simulink model "s06_sig_template_25"  (R2025b)
settings: Solver=ode4  StopTime=inf  FixedStep=P_sim_dt  EnableMultiTasking=on
InitFcn:
  | s06_data;
values from neighbouring files (symbols this model uses):
  P_c_locate_problist = ones(P_car_cnt, 1, 'single')    [s06_data.m]
  P_display_dt = 50e-3    (= 0.05)    [s06_data.m]
  P_dt = 25e-3    (= 0.025)    [s06_data.m]
  P_p_aMax = 1    [baseline_lqr_script.m]    (also in d71_data.m)
  P_p_Bf = 0.7    [d01_data.m]
  P_p_Br = 0.7    [d01_data.m]
  P_p_Cf = 2    [d01_data.m]
  P_p_Cr = 2    [d01_data.m]
  P_p_delta_max = 21.58/180*pi    (= 0.37664205258)    [d01_data.m]    (also in d71_data.m = 0.383972435439)
  P_p_deltan_max = 1    [d01_data.m]    (also in d71_data.m = 0.93)
  P_p_deltan_min = -P_p_deltan_max    (= -1)    [d01_data.m]    (also in d71_data.m = -0.93)
  P_p_Df = 2    [d01_data.m]
  P_p_Dr = 2.5    [d01_data.m]
  P_p_Ef = -0.1    [d01_data.m]
  P_p_EG = 0    [d01_data.m]    (also in d71_data.m = 0.02)
  P_p_Er = -0.05    [d01_data.m]
  P_p_J = 192e-6    (= 0.000192)    [d01_data.m]    (also in d71_data.m = 3e-06)
  P_p_k = 2.51    [d01_data.m]    (also in d71_data.m = 3.4)
  P_p_kd0 = 0.04    [d71_data.m]
  P_p_kd1 = 0.15    [d71_data.m]
  P_p_l = abs(P_p_frontaxle_1 + P_p_rearaxle_1)    [d01_data.m]    (also in d71_data.m = 0.0325)
  P_p_lf = P_p_frontaxle_1    (= 0.05)    [d01_data.m]    (also in d71_data.m = 0.01625)
  P_p_lr = P_p_rearaxle_1    (= 0.049)    [d01_data.m]    (also in d71_data.m = 0.01625)
  P_p_m = 132e-3    (= 0.132)    [d01_data.m]    (also in d71_data.m = 0.013)
  P_p_T = 316e-3    (= 0.316)    [d01_data.m]    (also in d71_data.m = 0.12)
  P_p_Tt = P_p_uTt + P_p_output_Tt    (= 0.11)    [d01_data.m]    (also in d71_data.m = 0.1)
  P_p_un_max = 1    [d01_data.m]    (also in d71_data.m = 0.2)
  P_p_un_min = -P_p_un_max    (= -1)    [d01_data.m]    (also in d71_data.m = -0.2)
  P_p_vRef = 0.2    [baseline_lqr_script.m]    (also in d71_data.m = 0.15)
  P_p_xvec0 = [ P_p_v0; P_p_s10; P_p_s20; P_p_psi0; 0; 0; 0 ]    [d01_data.m]    (also in d71_data.m)
  P_p_xvec1 = [ P_p_v0; P_p_s11; P_p_s21; P_p_psi1; 0; 0; 0 ]    [d01_data.m]    (also in d71_data.m)
  P_vfilter = single([ 0.0 0.0 ... (first row only)    [s06_data.m]
undefined symbols (not defined in the file or in its folder): CarInputsCmdForward, DiscIntNeverNeededParam, ManeuverTypePark, ManeuverTypePathFollow, mbc_car_display, P_cpseq, P_p, P_track
libraries: vrlib x2
(part 2 of 2)

== matlab function s06_sig_template_25/Car0/Motion Control/Feedback Pathfollowing ==
  data: v_star input; delta_e output; s_star input; psi_star input; s input; psi input; P_p_l parameter
function delta_e = fb_pf(v_star, s_star,psi_star,s,psi,P_p_l)
    %control deviation (see slideset 9 slide 13)
    sc2e=(s(2)-s_star(2))*cos(psi_star)-(s(1)-s_star(1))*sin(psi_star);
    % psi_e = psi - psi_star;
    % if abs(psi_e) < pi
    %     psi_e = -
    psi_e = atan2(sin(psi - psi_star), cos(psi - psi_star)); % wrapped psi_e=psi-psi_star
    
    Tw=0.175; %[s] time constant of pt1 dynamics

    %control law (see slideset 9 slide 20)
    % delta_e = -P_p_l*sc2e/(Tw^2 * v_star^2) - 2*P_p_l*psi_e/(Tw*v_star);

    v_min = 0.05;  % TODO: minimum effective speed, tune this
    v_eff = max(abs(v_star), v_min);

    delta_e = -P_p_l*sc2e/(Tw^2 * v_eff^2) ...
        -2*P_p_l*psi_e/(Tw*v_eff);

== matlab function s06_sig_template_25/Car0/Motion Control/MATLAB Function ==
  data: vRef output; k input; P_dt parameter; P_p_vRef parameter; P_p_aMax parameter
function vRef = generate_vRef(k, P_dt, P_p_vRef, P_p_aMax)
% Generate a discrete ramp speed reference.
%
% Inputs:
%   k          - discrete time index, integer: 0, 1, 2, ...
%   P_dt       - sample time [s]
%   P_p_vRef   - final target speed [m/s]
%   P_p_aMax   - maximum reference acceleration [m/s^2]
%
% Output:
%   vRef       - speed reference [m/s]

t = double(k) * P_dt;

vRef = P_p_aMax * t;

% Hold constant after reaching the target speed
vRef = min(vRef, P_p_vRef);

end

== matlab function s06_sig_template_25/Car0/Motion Control/performance monitor ==
  data: s_car input; psi_car input; SPLINE input; sc2e output; psiError output; progress output; simTime input; reset input; lapCount output; lapDone output; lapTimeLast output; lapIAELast output; lapRMSELast output; lapPsiRMSELast output
function [sc2e, psiError, progress, lapCount, lapDone, ...
          lapTimeLast, lapIAELast, lapRMSELast, ...
          lapPsiRMSELast] = ...
    performance_monitor(s_car, psi_car, SPLINE, simTime, reset)
% PERFORMANCE_MONITOR
% Independent path-following performance measurement.
%
% Inputs
%   s_car    : current vehicle position [x; y]
%   psi_car  : current vehicle heading angle [rad]
%   SPLINE   : MAD76 spline bus signal
%   simTime  : discrete simulation time [s]
%   reset    : reset monitor state
%
% Outputs
%   sc2e            : current signed lateral error [m]
%   psiError        : current wrapped heading error [rad]
%   progress        : accumulated progress in current lap [m]
%   lapCount        : number of completed laps
%   lapDone         : one-sample pulse when a lap is completed
%   lapTimeLast     : duration of last completed lap [s]
%   lapIAELast      : lateral-error IAE over last lap [m*s]
%   lapRMSELast     : lateral-error RMSE over last lap [m]
%   lapPsiRMSELast  : heading-error RMSE over last lap [rad]

persistent initialized
persistent previousArc
persistent previousTime
persistent accumulatedProgress
persistent lapStartTime

persistent lapIAE
persistent lapISE
persistent lapPsiISE

persistent completedLaps

persistent savedLapTime
persistent savedLapIAE
persistent savedLapRMSE
persistent savedLapPsiRMSE

%% Default outputs
sc2e           = 0.0;
psiError       = 0.0;
progress       = 0.0;
lapCount       = uint32(0);
lapDone        = false;
lapTimeLast    = 0.0;
lapIAELast     = 0.0;
lapRMSELast    = 0.0;
lapPsiRMSELast = 0.0;

%% Extract spline data
breakslen = int32(SPLINE.breakslen);
points    = SPLINE.points;
ppcoefs   = SPLINE.coefs;
periodic  = logical(SPLINE.periodic);

if breakslen <= 1
    return;
end

trackLength = double(points(1, breakslen));

if trackLength <= 0
    return;
end

%% Find nearest point on the reference spline
[arcPosition, nearestIndex] = mbc_spline_get_nearest( ...
    breakslen, ...
    points, ...
    ppcoefs, ...
    periodic, ...
    s_car, ...
    int32(1), ...
    breakslen);

%% Evaluate spline at nearest arc-length position
[s_ref, sd_ref, ~, ~] = mbc_ppval( ...
    breakslen, ...
    points(1,:), ...
    ppcoefs, ...
    arcPosition, ...
    nearestIndex);

%% Reference heading
psi_ref = double(atan2(sd_ref(2), sd_ref(1)));

%% Signed lateral error
normal_ref = [-sin(psi_ref);
               cos(psi_ref)];

position_error = ...
    double(s_car(1:2)) - double(s_ref(1:2));

sc2e = normal_ref.' * position_error;

%% Wrapped heading error
% Result is always between -pi and pi.
psiDifference = double(psi_car) - psi_ref;

psiError = atan2( ...
    sin(psiDifference), ...
    cos(psiDifference));

%% Initialization or external reset
if isempty(initialized) || reset
    initialized = true;

    previousArc         = double(arcPosition);
    previousTime        = double(simTime);
    accumulatedProgress = 0.0;
    lapStartTime        = double(simTime);

    lapIAE    = 0.0;
    lapISE    = 0.0;
    lapPsiISE = 0.0;

    completedLaps = uint32(0);

    savedLapTime    = 0.0;
    savedLapIAE     = 0.0;
    savedLapRMSE    = 0.0;
    savedLapPsiRMSE = 0.0;

    progress       = 0.0;
    lapCount       = completedLaps;
    lapTimeLast    = savedLapTime;
    lapIAELast     = savedLapIAE;
    lapRMSELast    = savedLapRMSE;
    lapPsiRMSELast = savedLapPsiRMSE;

    return;
end

%% Time increment
dt = double(simTime) - previousTime;

if dt < 0
    dt = 0.0;
end

%% Unwrap periodic arc-length increment
deltaArc = double(arcPosition) - previousArc;

if periodic
    if deltaArc < -0.5 * trackLength
        % Forward crossing from track end to track beginning
        deltaArc = deltaArc + trackLength;

    elseif deltaArc > 0.5 * trackLength
        % Backward crossing from track beginning to track end
        deltaArc = deltaArc - trackLength;
    end
end

accumulatedProgress = accumulatedProgress + deltaArc;

%% Accumulate error metrics
% Lateral IAE
lapIAE = lapIAE + abs(sc2e) * dt;

% Lateral ISE
lapISE = lapISE + sc2e^2 * dt;

% Heading-error ISE
lapPsiISE = lapPsiISE + psiError^2 * dt;

%% Detect completed lap
if accumulatedProgress >= trackLength
    currentLapTime = double(simTime) - lapStartTime;

    savedLapTime = currentLapTime;
    savedLapIAE  = lapIAE;

    if currentLapTime > 0
        savedLapRMSE = sqrt( ...
            lapISE / currentLapTime);

        savedLapPsiRMSE = sqrt( ...
            lapPsiISE / currentLapTime);
    else
        savedLapRMSE    = 0.0;
        savedLapPsiRMSE = 0.0;
    end

    completedLaps = completedLaps + uint32(1);
    lapDone = true;

    % Preserve progress beyond the finish line
    accumulatedProgress = ...
        accumulatedProgress - trackLength;

    % Start measuring the next lap
    lapStartTime = double(simTime);

    lapIAE    = 0.0;
    lapISE    = 0.0;
    lapPsiISE = 0.0;
end

%% Update persistent states
previousArc  = double(arcPosition);
previousTime = double(simTime);

%% Outputs
progress       = accumulatedProgress;
lapCount       = completedLaps;
lapTimeLast    = savedLapTime;
lapIAELast     = savedLapIAE;
lapRMSELast    = savedLapRMSE;
lapPsiRMSELast = savedLapPsiRMSE;

end

== matlab function s06_sig_template_25/Car0/Motion Control/Discrete-time Handler ==
  data: v input; k output; s input; psi input; v_k output; s_k output; psi_k output; Yp_k output
function [k, v_k, s_k, psi_k, Yp_k] = DiscreteTimeHandler(v, s, psi)

    persistent k_internal % discrete time index

    % initialize only once
    if isempty(k_internal)
        k_internal = -1;
    end

    % upon every incoming sample
    k_internal = k_internal + 1;

    % output
    k = k_internal;
    v_k = v; % this is to make sure the states we use later is consistent with the index
    s_k = s;
    psi_k = psi;

    %% integration for Yp
    persistent Yp_internal
    if isempty(Yp_internal)
        Yp_internal = 0;
    end
    
    Ts = 25e-3; % TODO: find the parameter in data.m
    Yp_internal = Yp_internal + double(v_k)*Ts;
    Yp_k = Yp_internal;

    %% NOTSURE: should we also initialize x0, v0 here? but in our case they
    % are just 0, right?

end

== matlab function s06_sig_template_25/Car0/Motion Control/SampledPositionReference ==
  data: wp input; k input; wp_k output; tE input
function wp_k = SampledPositionReference(wp, k, tE)
    
    Ts = 25e-3; % TODO: I really think we can find this parameter somewhere
    t = k*Ts;
    lap = 0;
    if t>tE
        lap = double(floor(t/tE));
        t = double(mod(t, tE));
    end
    wp_k = wp(6)*t^5 + wp(5)*t^4 + wp(4)*t^3 + wp(3)*t^2 + wp(2)*t + wp(1);
    wp_k = wp_k + lap * 2;
    % c5 = wp(6);
    % c4 = wp(5);
    % c3 = wp(4);
    % wp_k =-0.0008*t^4 + 0.0077 * t^3;
    % wp_k = c4*t^4 + c3*t^3;
    % 
    % if wp_k > 2
    %     wp_k = single(2);
    % end
    
end

== matlab function s06_sig_template_25/Car0/Motion Control/Position Feedforward Controller ==
  data: k input; uvp_k output; wp input; tE input
function uvp_k = PositionFeedFowardControl(k, wp, tE)

% analytical solution for feedforward signal 
% uvp(t) = Tw*wa(t+Tt)+wv(t+Tt)
    Ts = 25e-3;
    t=k*Ts;
    if t>tE
        t = double(mod(t, tE));
    end

    %t_t=t+P_p_Tt % for predicting deadtime when implemented

    Tw=0.2; %[s] time constant of pt1 dynamics
    c5=wp(6);
    c4=wp(5);
    c3=wp(4);
    c2=wp(3);
    c1=wp(2);
    wv=5*c5*t^4+4*c4*t^3+3*c3*t^2+2*c2*t+c1;
    wa=20*c5*t^3+12*c4*t^2+6*c3*t+2*c2;
    uvp_k=Tw*wa+wv;
end

== matlab function s06_sig_template_25/Car0/Motion Control/GP ==
  data: u input; y output; P_p_Tt parameter; P_dt parameter; P_p_T parameter; P_p_k parameter
function y = SmithPredictor(u, P_p_Tt, P_dt, P_p_T, P_p_k)
    % SMITH PREDICTOR IMPLEMENTATION
    % Calculates the difference between undelayed and delayed plant responses
   
    delay_steps = round(P_p_Tt / P_dt);
   
    if delay_steps < 1
        delay_steps = 1;
    end
   
    % MEMORY VARIABLES
    persistent y_undelayed_last
    persistent delay_buffer
   
    % INITIALIZATION
    if isempty(y_undelayed_last)
        y_undelayed_last = single(0);
        delay_buffer = zeros(delay_steps, 1, 'single');
    end
   
    % DYNAMIC BUFFER RESIZING
    if length(delay_buffer) ~= delay_steps
        new_buffer = zeros(delay_steps, 1, 'single');
        elements_to_copy = min(length(delay_buffer), delay_steps);
        new_buffer(1:elements_to_copy) = delay_buffer(1:elements_to_copy);
        delay_buffer = new_buffer;
    end
   
    % 1. UNDELAYED PLANT MODEL (Forward Euler)
    y_undelayed = y_undelayed_last + single(P_dt / P_p_T) * (single(P_p_k) * u - y_undelayed_last);
    % can try the exact
   
    % 2. DELAYED PLANT MODEL
    y_delayed = delay_buffer(end);
   
    % 3. BUFFER UPDATE
    if length(delay_buffer) > 1
        delay_buffer(2:end) = delay_buffer(1:end-1);
    end
    delay_buffer(1) = y_undelayed;
   
    % 4. OUTPUT
    y = single(y_undelayed - y_delayed);
   
    % SAVE STATE
    y_undelayed_last = y_undelayed;
end

== matlab function s06_sig_template_25/Car0/Motion Control/G_R1 ==
  data: e input; u output; e_last input; ui_last input; ui output; P_p_un_max parameter
function [u, ui] = pi_controller(e,e_last,ui_last,P_p_un_max)
   kr=0.177;
   Ti=0.12;
   ki=kr/Ti;
   T_sampling=0.025;
   
   up = kr*e;
   ui_increment = (T_sampling/2)*ki*(e+e_last);
   u_test = up + ui_last + ui_increment;

   if abs(u_test) > P_p_un_max
       u = P_p_un_max * sign(u_test);
       ui = ui_last;
   else
       u = u_test;
       ui = ui_last + ui_increment;
   end

   u = single(u);

== matlab function s06_sig_template_25/Car0/Motion Control/MATLAB Function1 ==
  data: sc2e input; psiError input; currentOK output; runOK output; un input; deltan input; lapDone input; reset input; runSuccessful output; trackOK output; inputRateOK output; maxAbsSc2e output; maxAbsPsiError output; maxAbsDun output; maxAbsDdeltan output; P_dt parameter; pedalEffortLast output; steeringEffortLast output
function [currentOK, runOK, runSuccessful, ...
          trackOK, inputRateOK, ...
          maxAbsSc2e, maxAbsPsiError, ...
          maxAbsDun, maxAbsDdeltan, ...
          pedalEffortLast, steeringEffortLast] = ...
    limit_check(sc2e, psiError, un, deltan, ...
                lapDone, reset, P_dt)
% LIMIT_CHECK
%
% Boolean convention:
%   1 = criterion satisfied
%   0 = criterion violated
%
% Inputs
%   sc2e      : signed lateral error [m]
%   psiError  : wrapped heading error [rad]
%   un        : normalized pedal command
%   deltan    : normalized steering command
%   lapDone   : one-sample pulse when one lap is completed
%   reset     : reset monitor
%   P_dt      : sample time [s]
%
% Outputs
%   currentOK          : current sample satisfies all checked limits
%   runOK              : no checked limit has been violated so far
%   runSuccessful      : completed lap with no checked violation
%   trackOK            : track boundary never violated
%   inputRateOK        : actuator rates never violated limits
%   maxAbsSc2e         : maximum absolute lateral error [m]
%   maxAbsPsiError     : maximum absolute heading error [rad]
%   maxAbsDun          : maximum pedal-command rate [1/s]
%   maxAbsDdeltan      : maximum steering-command rate [1/s]
%   pedalEffortLast    : integral of un^2 over last lap
%   steeringEffortLast : integral of deltan^2 over last lap

%% Limits
sc2eMax = 0.06;       % [m]

% Maximum normalized pedal-command rate
dunMax = 3.744;       % [1/s]

% Assumed physical steering speed:
% 3 rev/s = 6*pi rad/s
deltaMaxPhysical  = 0.3839;  % [rad]
ddeltaMaxPhysical = 6*pi;    % [rad/s]

% Convert physical steering rate to normalized steering-command rate
ddeltanMax = ddeltaMaxPhysical * 0.93 / deltaMaxPhysical;

% Numerical tolerance
tol = 1e-9;

%% Persistent states
persistent initialized
persistent previousUn
persistent previousDeltan

persistent trackOKStored
persistent inputRateOKStored

persistent lapCompletedStored
persistent runSuccessfulStored

persistent maxSc2eStored
persistent maxPsiErrorStored
persistent maxDunStored
persistent maxDdeltanStored

persistent pedalEffortAccumulated
persistent steeringEffortAccumulated
persistent savedPedalEffort
persistent savedSteeringEffort

%% Initialize or reset
if isempty(initialized) || reset
    initialized = true;

    previousUn     = double(un);
    previousDeltan = double(deltan);

    trackOKStored     = true;
    inputRateOKStored = true;

    lapCompletedStored  = false;
    runSuccessfulStored = false;

    maxSc2eStored     = abs(double(sc2e));
    maxPsiErrorStored = abs(double(psiError));
    maxDunStored      = 0.0;
    maxDdeltanStored  = 0.0;

    pedalEffortAccumulated    = 0.0;
    steeringEffortAccumulated = 0.0;

    savedPedalEffort    = 0.0;
    savedSteeringEffort = 0.0;

    currentOK     = true;
    runOK         = true;
    runSuccessful = false;

    trackOK     = true;
    inputRateOK = true;

    maxAbsSc2e          = maxSc2eStored;
    maxAbsPsiError      = maxPsiErrorStored;
    maxAbsDun           = maxDunStored;
    maxAbsDdeltan       = maxDdeltanStored;
    pedalEffortLast     = savedPedalEffort;
    steeringEffortLast  = savedSteeringEffort;

    return;
end

%% Calculate actuator rates
if P_dt > 0
    dt = double(P_dt);

    dun = ...
        (double(un) - previousUn) / dt;

    ddeltan = ...
        (double(deltan) - previousDeltan) / dt;
else
    dt = 0.0;

    dun     = inf;
    ddeltan = inf;
end

%% Current-sample checks
trackOKNow = ...
    abs(double(sc2e)) <= sc2eMax + tol;

inputRateOKNow = ...
    abs(dun)     <= dunMax     + tol && ...
    abs(ddeltan) <= ddeltanMax + tol;

currentOK = ...
    trackOKNow && inputRateOKNow;

%% Latch failures
trackOKStored = ...
    trackOKStored && trackOKNow;

inputRateOKStored = ...
    inputRateOKStored && inputRateOKNow;

%% Update maximum observed quantities
maxSc2eStored = max( ...
    maxSc2eStored, ...
    abs(double(sc2e)));

maxPsiErrorStored = max( ...
    maxPsiErrorStored, ...
    abs(double(psiError)));

maxDunStored = max( ...
    maxDunStored, ...
    abs(dun));

maxDdeltanStored = max( ...
    maxDdeltanStored, ...
    abs(ddeltan));

%% Accumulate quadratic control effort
if dt > 0
    pedalEffortAccumulated = ...
        pedalEffortAccumulated + double(un)^2 * dt;

    steeringEffortAccumulated = ...
        steeringEffortAccumulated + double(deltan)^2 * dt;
end

%% Overall run condition
runOK = ...
    trackOKStored && inputRateOKStored;

%% Detect lap completion
if lapDone
    lapCompletedStored  = true;
    runSuccessfulStored = runOK;

    savedPedalEffort = ...
        pedalEffortAccumulated;

    savedSteeringEffort = ...
        steeringEffortAccumulated;

    pedalEffortAccumulated    = 0.0;
    steeringEffortAccumulated = 0.0;
end

runSuccessful = ...
    lapCompletedStored && runSuccessfulStored;

%% Update previous values
previousUn     = double(un);
previousDeltan = double(deltan);

%% Outputs
trackOK     = trackOKStored;
inputRateOK = inputRateOKStored;

maxAbsSc2e         = maxSc2eStored;
maxAbsPsiError     = maxPsiErrorStored;
maxAbsDun          = maxDunStored;
maxAbsDdeltan      = maxDdeltanStored;
pedalEffortLast    = savedPedalEffort;
steeringEffortLast = savedSteeringEffort;

end

== matlab function s06_sig_template_25/Localization/Locate/ObsSpline/Reference and Deviations ==
  data: wxe output; s input; psi input; widxkm1 input int32; spline input; P_c_spline_range parameter; wx output; ws output; wkappa output; widx output; ey output; epsi output
function [ wxe, wx, ws, wkappa, widx, ey, epsi ] = fcn(s, psi, widxkm1, spline, P_c_spline_range)
%#codegen
wxe = spline.points(1, spline.breakslen);
if widxkm1 < int32(1)
    % first call
    irangemin = int32(1);
    irangemax = int32(spline.breakslen);
else
    irangemin = widxkm1 - P_c_spline_range;
    irangemax = widxkm1 + P_c_spline_range;
end
[ w , widx ] = mbc_spline_get_reference(s, spline.breakslen, spline.points, spline.coefs, spline.periodic, 0, 0, irangemin, irangemax);
wx = w(1);
wpsi = w(2);
ws = w(3:4);
wkappa = w(5);
ey = -sin(wpsi) * (s(1) - ws(1)) + cos(wpsi) * (s(2) - ws(2));
epsi = mod(psi - wpsi + pi, 2*pi) - pi;
end

== matlab function s06_sig_template_25/Maneuver1/Create Maneuver ==
  data: type input; vmax input; xref input; P_track parameter; P_cpseq parameter; maneuver output Bus: DRIVEMANEUVER size=1
function maneuver = create_maneuver(type, vmax, xref, P_track, P_cpseq)
%#codegen

track = P_track.center;

maneuver = struct( ...
    'vmax', vmax, ... 
    'type', type, ...
    'xref', xref, ...
    'lapCount', uint32(0), ...
    'disableLaneMonitor', false, ...
    'isnew', true, ...
    'breakslen', track.breakslen, ...
    'points', track.points, ...
    'coefs', track.coefs, ...
    'segments', zeros(1, length(track.points), 'uint32'), ...
    'periodic', true, ...
    'cpseq', P_cpseq);
end

== matlab function s06_sig_template_25/Localization/Locate/ObsSpline/wx derivative ==
  data: wx input; wxm1 input; xe input; wxd output; P_dt parameter
function wxd  = wx2wv(wx, wxm1, xe, P_dt)
wxd = single(0);
if wxm1 > -1
    wxd = (mod(wx - wxm1 + 0.5 * xe, xe) - 0.5 * xe) / P_dt;
end
end

== matlab function s06_sig_template_25/Maneuver0/Create Maneuver ==
  data: type input; vmax input; xref input; P_track parameter; P_cpseq parameter; maneuver output Bus: DRIVEMANEUVER size=1
function maneuver = create_maneuver(type, vmax, xref, P_track, P_cpseq)
%#codegen

track = P_track.center;

maneuver = struct( ...
    'vmax', vmax, ... 
    'type', type, ...
    'xref', xref, ...
    'lapCount', uint32(0), ...
    'disableLaneMonitor', false, ...
    'isnew', true, ...
    'breakslen', track.breakslen, ...
    'points', track.points, ...
    'coefs', track.coefs, ...
    'segments', zeros(1, length(track.points), 'uint32'), ...
    'periodic', true, ...
    'cpseq', P_cpseq);
end

== matlab function s06_sig_template_25/Localization/Locate/ObsSpline/Reference and Deviations1 ==
  data: wxe output; s input; psi input; widxkm1 input int32; spline input; P_c_spline_range parameter; w output; widx output; ey output; epsi output
function [ wxe, w, widx, ey, epsi ] = fcn(s, psi, widxkm1, spline, P_c_spline_range)
%#codegen
wxe = spline.points(1, spline.breakslen);
if widxkm1 < int32(1)
    % first call
    irangemin = int32(1);
    irangemax = int32(spline.breakslen);
else
    irangemin = widxkm1 - P_c_spline_range;
    irangemax = widxkm1 + P_c_spline_range;
end
[ w , widx ] = mbc_spline_get_reference(s, spline.breakslen, spline.points, spline.coefs, spline.periodic, 0, 0, irangemin, irangemax);
wpsi = w(2);
ws = w(3:4);
ey = -sin(wpsi) * (s(1) - ws(1)) + cos(wpsi) * (s(2) - ws(2));
epsi = mod(psi - wpsi + pi, 2*pi) - pi;
end

== matlab function s06_sig_template_25/Localization/Locate/ObsSpline/Reference and Deviations2 ==
  data: wxe output; s input; psi input; widxkm1 input int32; spline input; P_c_spline_range parameter; w output; widx output; ey output; epsi output
function [ wxe, w, widx, ey, epsi ] = fcn(s, psi, widxkm1, spline, P_c_spline_range)
%#codegen
wxe = spline.points(1, spline.breakslen);
if widxkm1 < int32(1)
    % first call
    irangemin = int32(1);
    irangemax = int32(spline.breakslen);
else
    irangemin = widxkm1 - P_c_spline_range;
    irangemax = widxkm1 + P_c_spline_range;
end
[ w , widx ] = mbc_spline_get_reference(s, spline.breakslen, spline.points, spline.coefs, spline.periodic, 0, 0, irangemin, irangemax);
wpsi = w(2);
ws = w(3:4);
ey = -sin(wpsi) * (s(1) - ws(1)) + cos(wpsi) * (s(2) - ws(2));
epsi = mod(psi - wpsi + pi, 2*pi) - pi;
end
